simulink model "mass_spring_damper_animation"  (R2015a)
settings: Solver=ode45  StartTime=0.0  StopTime=inf  RelTol=1e-3
undefined symbols (not defined in the file or in its folder): drawMassSpringDamper
libraries: simulink x1
settings Model: Creator=ecestudent  LastModifiedBy=ecestudent

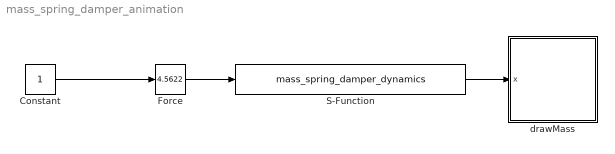
== system mass_spring_damper_animation ==
  Constant : Constant
  Force : simulink/Math Operations/Slider Gain  low=-10  gain=4.5622  high=10
  S-Function : S-Function  FunctionName=mass_spring_damper_dynamics  Parameters=AP
  drawMass : Subsystem
      mask Display: image(imread('tv.jpg'))
  wires:
  Constant/1 -> Force/1
  Force/1 -> S-Function/1
  S-Function/1 -> drawMass/1(x)

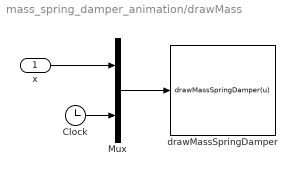
== system mass_spring_damper_animation/drawMass ==
  x : Inport
  Clock : Clock
  Mux : Mux  Inputs=2
  drawMassSpringDamper : MATLABFcn  MATLABFcn=drawMassSpringDamper(u)  OutputDimensions=0
      mask Display: image(imread('tv.jpg'))
  wires:
  x/1 -> Mux/1
  Clock/1 -> Mux/2
  Mux/1 -> drawMassSpringDamper/1
